simulink library "Power_Shaft3_Ideal_A1_L2_R2"  (R2023a)
settings: Solver=VariableStepAuto  StartTime=0.0  StopTime=10.0  RelTol=1e-3
undefined symbols (not defined in the file): ShaftA1, ShaftL2, ShaftR2
libraries: fl_lib x4, Power_Components x3, nesl_utility x3, sm_lib x1
Description:
  | Component of Simscape Vehicle Templates Library
  | 
  | Copyright 2018-2024 The MathWorks, Inc.
settings Model: Creator=smiller  LastModifiedBy=smiller
settings SolverCC: AlgebraicLoopSolver=TrustRegion
settings DataIOCC: ReturnWorkspaceOutputs=off
settings DebuggingCC: UnconnectedInputMsg=warning  UnconnectedOutputMsg=warning  UnconnectedLineMsg=warning  ArithmeticOperatorsInVariantConditions=warning
settings ModelReferenceCC: EnableRefExpFcnMdlSchedulingChecks=on
settings SFSimCC: CustomCodeUndefinedFunction=UseInterfaceOnly
settings RTWCC: DLArmComputeVersion=19.05

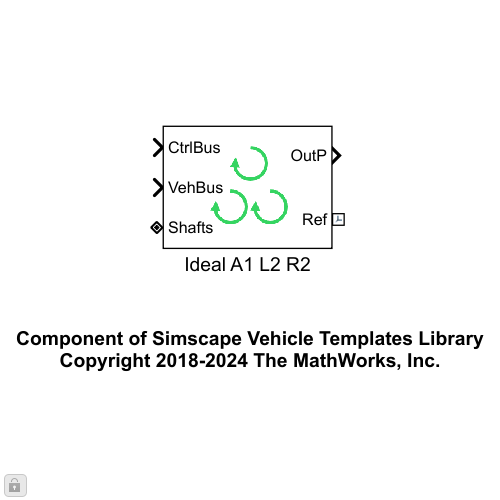
[thumbnail: Simulink's stored preview of the top-level diagram]
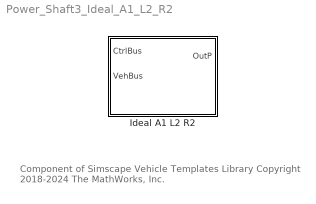
== system Power_Shaft3_Ideal_A1_L2_R2 ==
  note: Component of Simscape Vehicle Templates Library
      | Copyright 2018-2024 The MathWorks, Inc.
  Ideal A1 L2 R2 : Subsystem  VariantControl=IdealTwoMotor  mask(Three Ideal Motors, Axle 1, Left Axle 2, Right Axle 2){motor_ts_a1=100, motor_ts_l2=100, motor_ts_r2=100}
      mask prompts: motor_ts_a1 "Axle 1 Motor Cutoff Frequency (Hz)"; motor_ts_l2 "Wheel L2 Motor Cutoff Frequency (Hz)"; motor_ts_r2 "Wheel R2 Motor Cutoff Frequency (Hz)"
      mask help: Models three ideal motors connected to a differential for the front axle and directly to the wheels on the rear axle.
      mask Display: image('sm_car_vehicle_power_i3motor_A1L2R2_IMAGE.png');

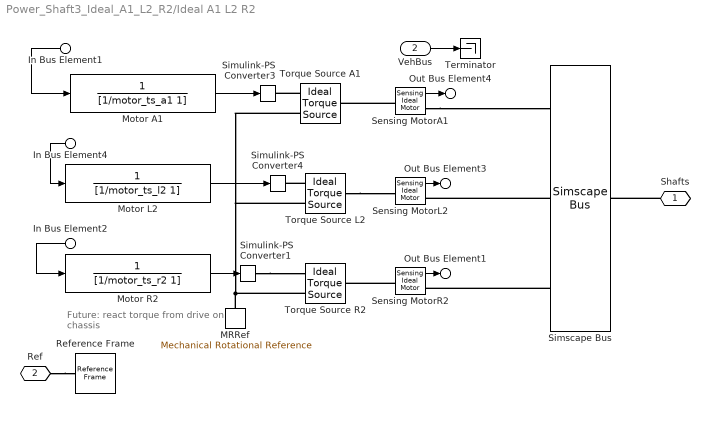
== system Power_Shaft3_Ideal_A1_L2_R2/Ideal A1 L2 R2 ==
  note: Future: react torque from
      | drive on chassis
  In Bus Element1 : Inport  PortName=CtrlBus  Element=MMotorA1Demand
  In Bus Element2 : Inport  PortName=CtrlBus  Element=MMotorR2Demand
  In Bus Element4 : Inport  PortName=CtrlBus  Element=MMotorL2Demand
  VehBus : Inport  Port=2
  MRRef : fl_lib/Mechanical/Rotational Elements/Mechanical Rotational Reference
  Motor A1 : TransferFcn  Denominator=[1/motor_ts_a1 1]
  Motor L2 : TransferFcn  Denominator=[1/motor_ts_l2 1]
  Motor R2 : TransferFcn  Denominator=[1/motor_ts_r2 1]
  Reference Frame : sm_lib/Frames and Transforms/Reference Frame
  Sensing MotorA1 : Power_Components/Sensing Ideal Motor  SystemSampleTime=-1  VariantActivationTime=update diagram  Latency=0  AutoFrameSizeCalculation=off
  Sensing MotorL2 : Power_Components/Sensing Ideal Motor  SystemSampleTime=-1  VariantActivationTime=update diagram  Latency=0  AutoFrameSizeCalculation=off
  Sensing MotorR2 : Power_Components/Sensing Ideal Motor  SystemSampleTime=-1  VariantActivationTime=update diagram  Latency=0  AutoFrameSizeCalculation=off
  Simscape Bus : SimscapeBus  HierarchyStrings=ShaftA1;ShaftL2;ShaftR2
  Simulink-PS Converter1 : nesl_utility/Simulink-PS Converter  PhysicalDomain=network_engine_domain  SubClassName=ps_input  LeftPortType=input  RightPortType=output  PseudoPeriodic=off  Frequencies=[]  NoiseDistribution=none  NoiseParameters=[]  Unit=1  AffineConversion=off  FilteringAndDerivatives=provide  SimscapeFilterOrder=1  InputFilterTimeConstant=0.001  UdotUserProvided=0
  Simulink-PS Converter3 : nesl_utility/Simulink-PS Converter  PhysicalDomain=network_engine_domain  SubClassName=ps_input  LeftPortType=input  RightPortType=output  PseudoPeriodic=off  Frequencies=[]  NoiseDistribution=none  NoiseParameters=[]  Unit=1  AffineConversion=off  FilteringAndDerivatives=provide  SimscapeFilterOrder=1  InputFilterTimeConstant=0.001  UdotUserProvided=0
  Simulink-PS Converter4 : nesl_utility/Simulink-PS Converter  PhysicalDomain=network_engine_domain  SubClassName=ps_input  LeftPortType=input  RightPortType=output  PseudoPeriodic=off  Frequencies=[]  NoiseDistribution=none  NoiseParameters=[]  Unit=1  AffineConversion=off  FilteringAndDerivatives=provide  SimscapeFilterOrder=1  InputFilterTimeConstant=0.001  UdotUserProvided=0
  Terminator : Terminator
  Torque Source A1 : fl_lib/Mechanical/Mechanical Sources/Ideal Torque Source
  Torque Source L2 : fl_lib/Mechanical/Mechanical Sources/Ideal Torque Source
  Torque Source R2 : fl_lib/Mechanical/Mechanical Sources/Ideal Torque Source
  Shafts : PMIOPort  Side=Left
  Ref : PMIOPort  Port=2  Side=Right
  Out Bus Element4 : Outport  VectorParamsAs1DForOutWhenUnconnected=off  PortName=OutP  Element=MotorA1
  Out Bus Element3 : Outport  VectorParamsAs1DForOutWhenUnconnected=off  PortName=OutP  Element=MotorL2
  Out Bus Element1 : Outport  VectorParamsAs1DForOutWhenUnconnected=off  PortName=OutP  Element=MotorR2
  wires:
  Motor A1/1 -> Simulink-PS Converter3/1
  In Bus Element1/1 -> Motor A1/1
  VehBus/1 -> Terminator/1
  Sensing MotorA1/1 -> Out Bus Element4/1
  Motor R2/1 -> Simulink-PS Converter1/1
  Motor L2/1 -> Simulink-PS Converter4/1
  Sensing MotorL2/1 -> Out Bus Element3/1
  Sensing MotorR2/1 -> Out Bus Element1/1
  In Bus Element2/1 -> Motor R2/1
  In Bus Element4/1 -> Motor L2/1
  connections:
  Sensing MotorA1/RConn1 -- Simscape Bus/LConn1
  Ref/RConn1 -- Reference Frame/RConn1
  Shafts/RConn1 -- Simscape Bus/RConn1
  Torque Source A1/RConn1 -- Simulink-PS Converter3/RConn1
  Sensing MotorA1/LConn1 -- Torque Source A1/LConn1
  Torque Source R2/RConn2 -- Torque Source L2/RConn2 -- Torque Source A1/RConn2 -- MRRef/LConn1
  Torque Source L2/RConn1 -- Simulink-PS Converter4/RConn1
  Simscape Bus/LConn3 -- Sensing MotorR2/RConn1
  Torque Source L2/LConn1 -- Sensing MotorL2/LConn1
  Simscape Bus/LConn2 -- Sensing MotorL2/RConn1
  Simulink-PS Converter1/RConn1 -- Torque Source R2/RConn1
  Sensing MotorR2/LConn1 -- Torque Source R2/LConn1
